simulink model "Troubleshooting_Engine_v5"  (R2013a)
settings: Solver=ode3  StartTime=0.0  StopTime=500  FixedStep=0.25  RelTol=1e-3
undefined symbols (not defined in the file or in its folder): sigbuilder_block
settings Model: Creator=Raymond  LastModifiedBy=Raymond

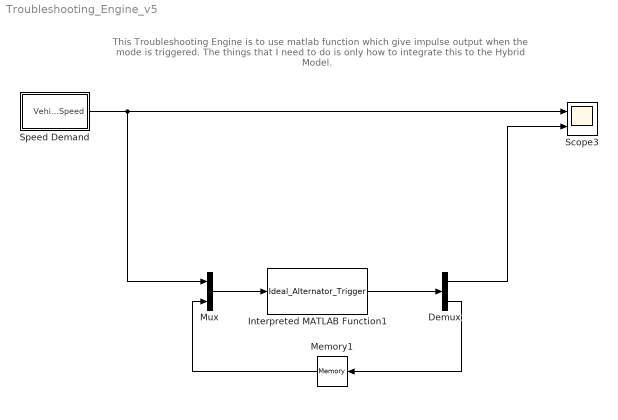
== system Troubleshooting_Engine_v5 ==
  note: This Troubleshooting Engine is to use matlab function
      | which give impulse output when the mode is triggered.
      | The things that I need to do is only how to integrate this to the Hybrid Model.
  Demux : Demux  Outputs=2
  Interpreted MATLAB Function1 : MATLABFcn  MATLABFcn=Ideal_Alternator_Trigger
  Memory1 : Memory
  Mux : Mux  Inputs=2
  Scope3 : Scope  NumInputPorts=2
      settings: YMin=-5~-5  YMax=5~5
  Speed Demand : Subsystem
      mask Display: disp('DriveCycle')
  wires:
  Speed Demand/1(VehicleSpeed) -> Scope3/1, Mux/1
  Interpreted MATLAB Function1/1 -> Demux/1
  Demux/2 -> Memory1/1
  Mux/1 -> Interpreted MATLAB Function1/1
  Memory1/1 -> Mux/2
  Demux/1 -> Scope3/2

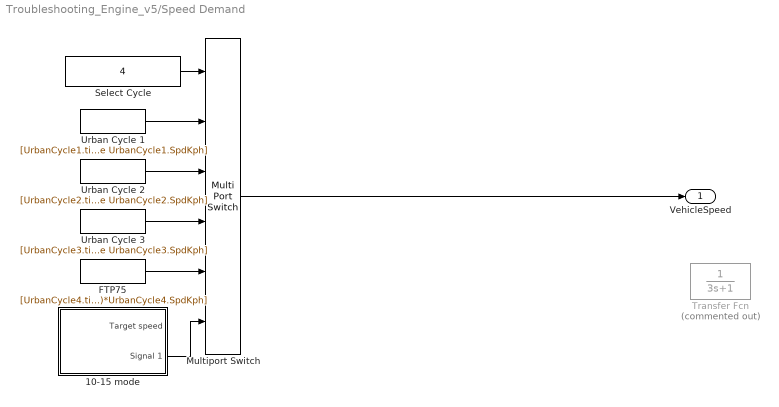
== system Troubleshooting_Engine_v5/Speed Demand ==
  "10-15 mode " : Subsystem  Tag=STV Subsys  LoadFcn=sigbuilder_block('load');  StartFcn=sigbuilder_block('start');  StopFcn=sigbuilder_block('stop');  ClipboardFcn=sigbuilder_block('clipboard');  mask(Sigbuilder block){}
      mask help: Sigbuilder GUI
      mask init:
      | if ~strcmp(get_param(bdroot(gcbh),'SimulationStatus'),'stopped') tuvar = sigbuilder_block('maskInit'); end
      settings: CopyFcn=sigbuilder_block('copy');  DeleteFcn=sigbuilder_block('delete');  ModelCloseFcn=sigbuilder_block('modelClose');  PreSaveFcn=sigbuilder_block('preSave');  PauseFcn=sigbuilder_block('pause')  ContinueFcn=sigbuilder_block('continue')  NameChangeFcn=sigbuilder_block('namechange');  OpenFcn=sigbuilder_block('open',[5.58621 35.3793 980.69 465.517 ]);  CloseFcn=sigbuilder_block('close');
      mask Display: plot(0,0,100,100,[10,10,40,40,10],[80,20,20,80,80],[40,10],[50,50], [40,27,10],[65,72,56],[40,25,25,10],[28,28,43,43]);
  FTP75 : FromWorkspace  VariableName=[UrbanCycle4.time Vehicle_MaxSpeed_kph/max(UrbanCycle4.SpdKph)*UrbanCycle4.SpdKph]  SampleTime=0
  Multiport Switch : MultiPortSwitch  Inputs=5
  Select Cycle : Constant  Value=4
  Transfer Fcn : TransferFcn  Commented=on  Denominator=[3 1]
  Urban Cycle 1 : FromWorkspace  VariableName=[UrbanCycle1.time UrbanCycle1.SpdKph]  SampleTime=0
  Urban Cycle 2 : FromWorkspace  VariableName=[UrbanCycle2.time UrbanCycle2.SpdKph]  SampleTime=0
  Urban Cycle 3 : FromWorkspace  VariableName=[UrbanCycle3.time UrbanCycle3.SpdKph]  SampleTime=0
  VehicleSpeed : Outport
  wires:
  Urban Cycle 3/1 -> Multiport Switch/4
  Select Cycle/1 -> Multiport Switch/1
  Urban Cycle 2/1 -> Multiport Switch/3
  Urban Cycle 1/1 -> Multiport Switch/2
  FTP75/1 -> Multiport Switch/5
  "10-15 mode "/2(Signal 1) -> Multiport Switch/6
  Multiport Switch/1 -> VehicleSpeed/1

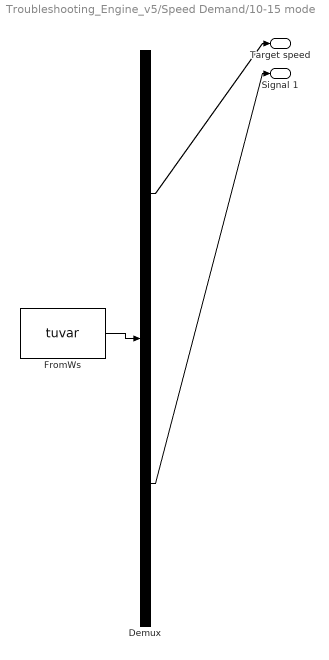
== system Troubleshooting_Engine_v5/Speed Demand/10-15 mode  ==
  Demux : Demux  Tag=STV Demux  Outputs=2
  FromWs : FromWorkspace  Tag=STV FromWs  VariableName=tuvar  SampleTime=0
      SigBuilderData=|
      | common.afterFinalStr = 'Extrapolate'
      | common.sampleTime = '0'
      | dataSet.timeRange = [0 660]
      | dataSet.name = '10-15 Mode Cycle'
      | sbobj.Groups.Name = '10-15 Mode Cycle'
      | sbobj.Groups.Signals(1).Name = 'Target speed'
      | sbobj.Groups.Signals(1).XData = [0 44 51 73 73 89 103 118 128 130 142 152 159 179 186 201 208 224 238 253 263 265 277 287 294 314 321 336 343 359 373 388 398 400 412 422 429 494 512 524 528 532 548 558 569 579 589 593 615 620 640 650 660]
      | sbobj.Groups.Signals(1).YData = [0 0 10 10 0 0 40 40 20 20 40 20 0 0 20 20 0 0 40 40 20 20 40 20 0 0 20 20 0 0 40 40 20 20 40 20 0 0 50 50 40 40 60 60 70 70 50 50 70 70 30 0 0]
      | sbobj.Groups.Signals(2).Name = 'Signal 1'
      | sbobj.Groups.Signals(2).XData = [0 20 120 120 220 220 320 320 420 420 520 520 620 650 660]
      | sbobj.Groups.Signals(2).YData = [0 10 10 20 20 30 30 40 39.8 50 50 60 60 0.5 0]
  Target speed : Outport  Tag=STV Outport
  Signal 1 : Outport  Tag=STV Outport  Port=2
  wires:
  FromWs/1 -> Demux/1
  Demux/1 -> Target speed/1
  Demux/2 -> Signal 1/1
